simulink model "all_test"  (R2023a)
settings: Solver=VariableStepAuto  StartTime=0.0  StopTime=Tf  RelTol=1e-3
values from neighbouring files (symbols this model uses):
  vehicle_data = getVehicleDataStruct()    [main.m]
undefined symbols (not defined in the file or in its folder): input
libraries: autolibshared x5
settings Model: Creator=ashkan  LastModifiedBy=ashkan

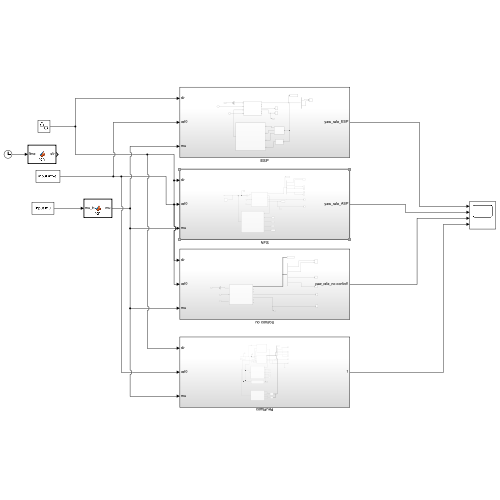
[thumbnail: Simulink's stored preview of the top-level diagram]
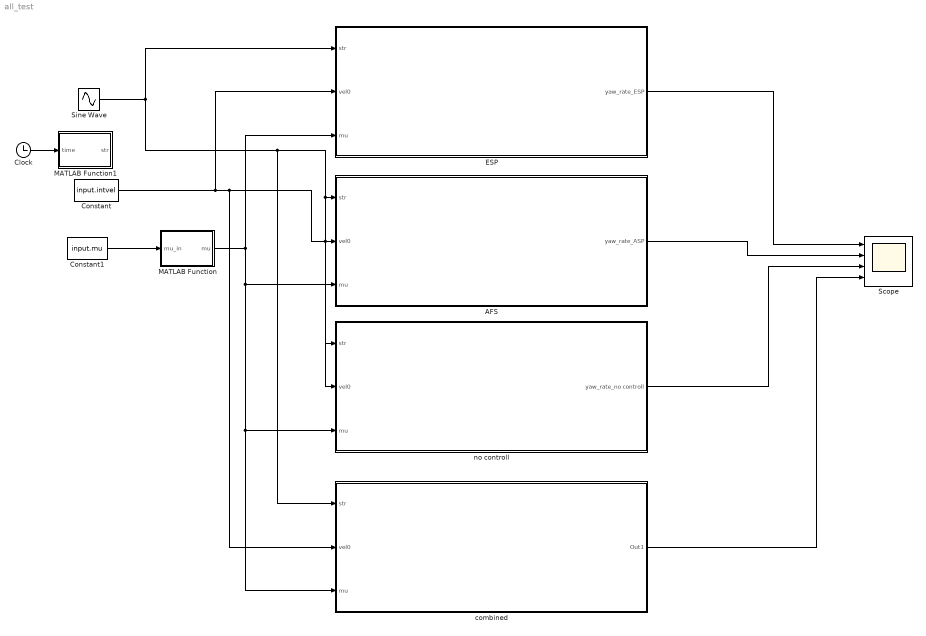
== system all_test ==
  AFS : Subsystem
  Clock : Clock
  Constant : Constant  Value=input.intvel
  Constant1 : Constant  Value=input.mu
  ESP : Subsystem
  MATLAB Function : MATLAB Function  TreatAsAtomicUnit=on
  MATLAB Function1 : MATLAB Function  TreatAsAtomicUnit=on
  Scope : Scope  NumInputPorts=4
  Sine Wave : Sin  Amplitude=input.str.amp  Frequency=input.str.freq  SampleTime=input.str.sample_time
  combined : Subsystem
  no controll : Subsystem
  wires:
  Constant/1 -> combined/2(vel0), no controll/2(vel0), AFS/2(vel0), ESP/2(vel0)
  Constant1/1 -> MATLAB Function/1(mu_in)
  Sine Wave/1 -> combined/1(str), no controll/1(str), AFS/1(str), ESP/1(str)
  MATLAB Function/1(mu) -> ESP/3(mu), AFS/3(mu), combined/3(mu), no controll/3(mu)
  ESP/1(yaw_rate_ESP) -> Scope/1
  AFS/1(yaw_rate_ASP) -> Scope/2
  no controll/1(yaw_rate_no controll) -> Scope/3
  Clock/1 -> MATLAB Function1/1(time)
  combined/1(Out1) -> Scope/4

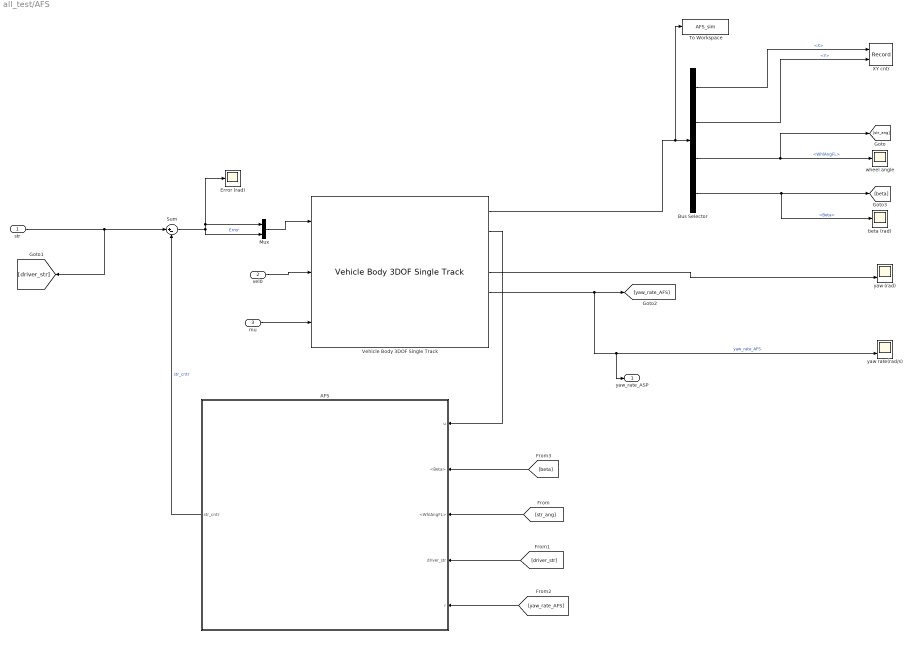
== system all_test/AFS ==
  str : Inport
  vel0 : Inport  Port=2
  mu : Inport  Port=3
  AFS : Subsystem
  Bus Selector : BusSelector  OutputSignals=InertFrm.Cg.Disp.X,InertFrm.Cg.Disp.Y,BdyFrm.FrntAxl.Steer.WhlAngFL,BdyFrm.Cg.Ang.Beta
  Error (rad) : Scope
  Mux : Mux  Inputs=2
  Sum : Sum  Inputs=|+-
  To Workspace : ToWorkspace  VariableName=AFS_sim  SaveFormat=Timeseries  SampleTime=-1
  Vehicle Body 3DOF Single Track : autolibshared/Vehicle Body 3DOF Single Track  trackMode=Dual  inputMode=External longitudinal velocity  frontSteerMode=on  rearSteerMode=off  windMode=off  muMode=on  extFMode=off  extMMode=off  htchFMode=off  htchMMode=off  extXo=off  extpsio=off  extxdoto=off  extro=off  extYo=off  extTamb=off  extydoto=off  aMode=2  NF=2  NR=2  m=vehicle_data.vehicle.m  a=vehicle_data.vehicle.Lf  b=vehicle_data.vehicle.Lr  h=vehicle_data.vehicle.hGs  dh=1  hh=0.2  X_o=0  xdot_o=0  CalphaMode=off  sigmaMode=off  d=0  hl=0  w="[vehicle_data.vehicle.Wf ,  vehicle_data.vehicle.Wr]"  Cy_f=vehicle_data.front_suspension.Ks_f  Cy_r=vehicle_data.rear_suspension.Ks_r  sigma_f=.1  sigma_r=.1  alpha_f_brk=[-.1 .1]  Cy_f_data=[-9e3 9e3]  alpha_r_brk=[-.1 .1]  Cy_r_data=[-9e3 9e3]  Y_o=0  ydot_o=0  Izz=4000  psi_o=0  r_o=0  Af=2  Cd=.3  Cl=.1  Cpm=.1  beta_w=[0 0.01:0.01:0.3]  Cs=[0 0.01:0.01:0.3]  Cym=[0 1e-6:0.01:0.3]  Pabs=101325  Tair=273  g=9.81  mu=1  xdot_tol=.01  Fznom=5000  Fxtire_sat=7e4  Fytire_sat=7e4  longOff=0  latOff=0  vertOff=0  wrapAng=off
  XY cntr : Record  FileSettingsInternal="{\"entries\":[{\"content\":{\"excelSettings\":{\"content\":{},\"type\":\"Streamout.ExcelSettings\"}},\"type\":\"Streamout.FileSettingStorage\",\"uuid\":\"\"}],\"packageUris\":[\"http:\\/\\/schema.mathworks.com\\/mf0\\/streamout_blocks\\/R2020a\"],\"version\":\"1.0\"}"  Layout=[1 1]  SignalsInternal="{\"entries\":[{\"content\":{\"signals\":[{\"content\":{\"blockPath\":[],\"dimensions\":[1],\"domain\":\"\",\"lineColor\":\"#22b573\",\"plots\":[1],\"port\":1,\"sid\":[\"\"],\"signalID\":22727,\"signalName\":\"<X>\"},\"type\":\"RecordBlkView.Signal\",\"uuid\":\"\"},{\"content\":{\"blockPath\":[],\"dimensions\":[1],\"domain\":\"\",\"lineColor\":\"#0072bd\",\"plots\":[1],\"port\":2,\"sid\":[\"\"],\"signalID\":22731,\"signalName\":\"<Y>\"},\"type\":\"RecordBlkView.Signal\",\"uuid\":\"\"}]},\"type\":\"RecordBlkView.InputSignals\",\"uuid\":\"\"}],\"packageUris\":[\"http:\\/\\/schema.mathworks.com\\/mf0\\/streamout_blocks\\/R2020a\"],\"version\":\"1.0\"}"  VisualizationBindings="{\"xyplotplugin\":{\"info\":[{\"series\":[{\"bindingParametersList\":[{\"parameter\":\"X-Axis\",\"signalID\":22727,\"signalName\":\"<X>\"},{\"parameter\":\"Y-Axis\",\"signalID\":22731,\"signalName\":\"<Y>\"}],\"seriesID\":47189}],\"subplotID\":1}]}}"  CompatibilityTag=XY
  beta (rad) : Scope
  wheel angle : Scope
  yaw (rad) : Scope  NumInputPorts=2
  yaw rate(rad/s) : Scope  NumInputPorts=2
  yaw_rate_ASP : Outport
  wires:
  Bus Selector/1 -> XY cntr/1  "<X>"
  [yaw_rate_AFS] -> AFS/5(r)
  Bus Selector/4 -> [beta], beta (rad)/1  "<Beta>"
  Bus Selector/3 -> [str_ang], wheel angle/1  "<WhlAngFL>"
  AFS/1(str_cntr) -> Sum/2  "str_cntr"
  Bus Selector/2 -> XY cntr/2  "<Y>"
  [str_ang] -> AFS/3(<WhlAngFL>)
  Vehicle Body 3DOF Single Track/5 -> [yaw_rate_AFS], yaw_rate_ASP/1, yaw rate(rad/s)/2  "yaw_rate_AFS"
  [driver_str] -> AFS/4(driver_str)
  str/1 -> [driver_str], Sum/1
  [beta] -> AFS/2(<Beta>)
  Sum/1 -> Mux/2, Mux/1, Error (rad)/1  "Error"
  Vehicle Body 3DOF Single Track/4 -> yaw (rad)/2
  Mux/1 -> Vehicle Body 3DOF Single Track/1
  Vehicle Body 3DOF Single Track/1 -> To Workspace/1, Bus Selector/1
  Vehicle Body 3DOF Single Track/2 -> AFS/1(u)
  vel0/1 -> Vehicle Body 3DOF Single Track/2
  mu/1 -> Vehicle Body 3DOF Single Track/3

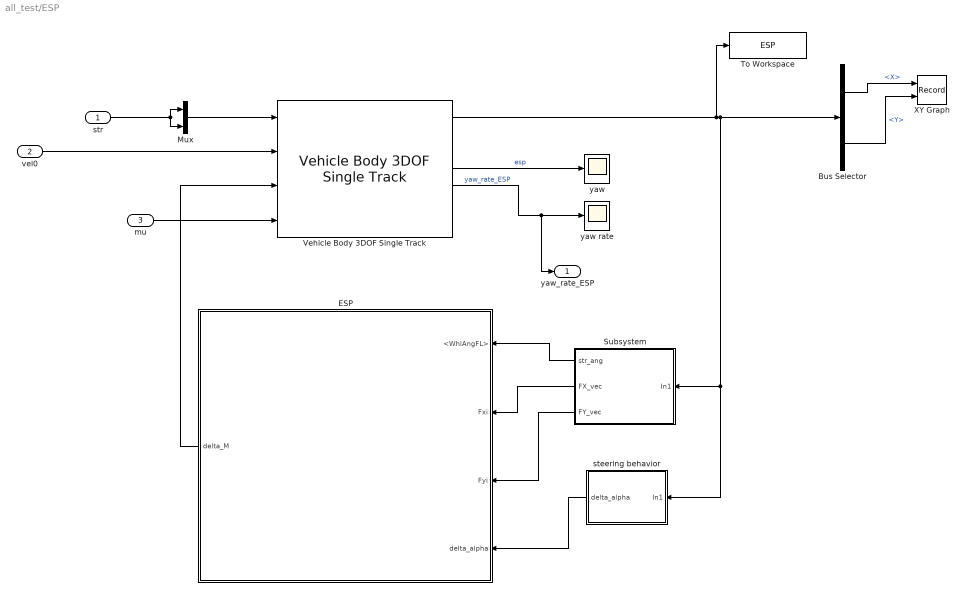
== system all_test/ESP ==
  str : Inport
  vel0 : Inport  Port=2
  mu : Inport  Port=3
  Bus Selector : BusSelector  OutputSignals=InertFrm.Cg.Disp.X,InertFrm.Cg.Disp.Y
  ESP : Subsystem
  Mux : Mux  Inputs=2
  Subsystem : Subsystem
  To Workspace : ToWorkspace  VariableName=ESP  SaveFormat=Timeseries  SampleTime=-1
  Vehicle Body 3DOF Single Track : autolibshared/Vehicle Body 3DOF Single Track  trackMode=Dual  inputMode=External longitudinal velocity  frontSteerMode=on  rearSteerMode=off  windMode=off  muMode=on  extFMode=off  extMMode=on  htchFMode=off  htchMMode=off  extXo=off  extpsio=off  extxdoto=off  extro=off  extYo=off  extTamb=off  extydoto=off  aMode=2  NF=2  NR=2  m=vehicle_data.vehicle.m  a=vehicle_data.vehicle.Lf  b=vehicle_data.vehicle.Lr  h=vehicle_data.vehicle.hGs  dh=1  hh=0.2  X_o=0  xdot_o=0  CalphaMode=off  sigmaMode=off  d=0  hl=0  w="[vehicle_data.vehicle.Wf ,  vehicle_data.vehicle.Wr]"  Cy_f=vehicle_data.front_suspension.Ks_f  Cy_r=vehicle_data.rear_suspension.Ks_r  sigma_f=.1  sigma_r=.1  alpha_f_brk=[-.1 .1]  Cy_f_data=[-9e3 9e3]  alpha_r_brk=[-.1 .1]  Cy_r_data=[-9e3 9e3]  Y_o=0  ydot_o=0  Izz=4000  psi_o=0  r_o=0  Af=2  Cd=.3  Cl=.1  Cpm=.1  beta_w=[0 0.01:0.01:0.3]  Cs=[0 0.01:0.01:0.3]  Cym=[0 1e-6:0.01:0.3]  Pabs=101325  Tair=273  g=9.81  mu=1  xdot_tol=.01  Fznom=5000  Fxtire_sat=7e4  Fytire_sat=7e4  longOff=0  latOff=0  vertOff=0  wrapAng=off
  XY Graph : Record  FileSettingsInternal="{\"entries\":[{\"content\":{\"excelSettings\":{\"content\":{},\"type\":\"Streamout.ExcelSettings\"}},\"type\":\"Streamout.FileSettingStorage\",\"uuid\":\"\"}],\"packageUris\":[\"http:\\/\\/schema.mathworks.com\\/mf0\\/streamout_blocks\\/R2020a\"],\"version\":\"1.0\"}"  Layout=[1 1]  SignalsInternal="{\"entries\":[{\"content\":{\"signals\":[{\"content\":{\"blockPath\":[],\"dimensions\":[1],\"domain\":\"\",\"lineColor\":\"#b746ff\",\"port\":1,\"sid\":[\"\"],\"signalID\":23776,\"signalName\":\"<X>\"},\"type\":\"RecordBlkView.Signal\",\"uuid\":\"\"},{\"content\":{\"blockPath\":[],\"dimensions\":[1],\"domain\":\"\",\"lineColor\":\"#64d413\",\"port\":2,\"sid\":[\"\"],\"signalID\":23780,\"signalName\":\"<Y>\"},\"type\":\"RecordBlkView.Signal\",\"uuid\":\"\"}]},\"type\":\"RecordBlkView.InputSignals\",\"uuid\":\"\"}],\"packageUris\":[\"http:\\/\\/schema.mathworks.com\\/mf0\\/streamout_blocks\\/R2020a\"],\"version\":\"1.0\"}"  VisualizationBindings="{\"xyplotplugin\":{\"info\":[{\"series\":[],\"subplotID\":1}]}}"  CompatibilityTag=XY
  steering behavior : Subsystem
  yaw : Scope
  yaw rate : Scope
  yaw_rate_ESP : Outport
  wires:
  Bus Selector/2 -> XY Graph/2  "<Y>"
  vel0/1 -> Vehicle Body 3DOF Single Track/2
  Vehicle Body 3DOF Single Track/1 -> To Workspace/1, Subsystem/1(In1), steering behavior/1(In1), Bus Selector/1
  Subsystem/2(FX_vec) -> ESP/2(Fxi)
  Subsystem/3(FY_vec) -> ESP/3(Fyi)
  Vehicle Body 3DOF Single Track/4 -> yaw/1  "esp"
  Vehicle Body 3DOF Single Track/5 -> yaw_rate_ESP/1, yaw rate/1  "yaw_rate_ESP"
  ESP/1(delta_M) -> Vehicle Body 3DOF Single Track/3
  mu/1 -> Vehicle Body 3DOF Single Track/4
  Subsystem/1(str_ang) -> ESP/1(<WhlAngFL>)
  Bus Selector/1 -> XY Graph/1  "<X>"
  str/1 -> Mux/1, Mux/2
  Mux/1 -> Vehicle Body 3DOF Single Track/1
  steering behavior/1(delta_alpha) -> ESP/4(delta_alpha)

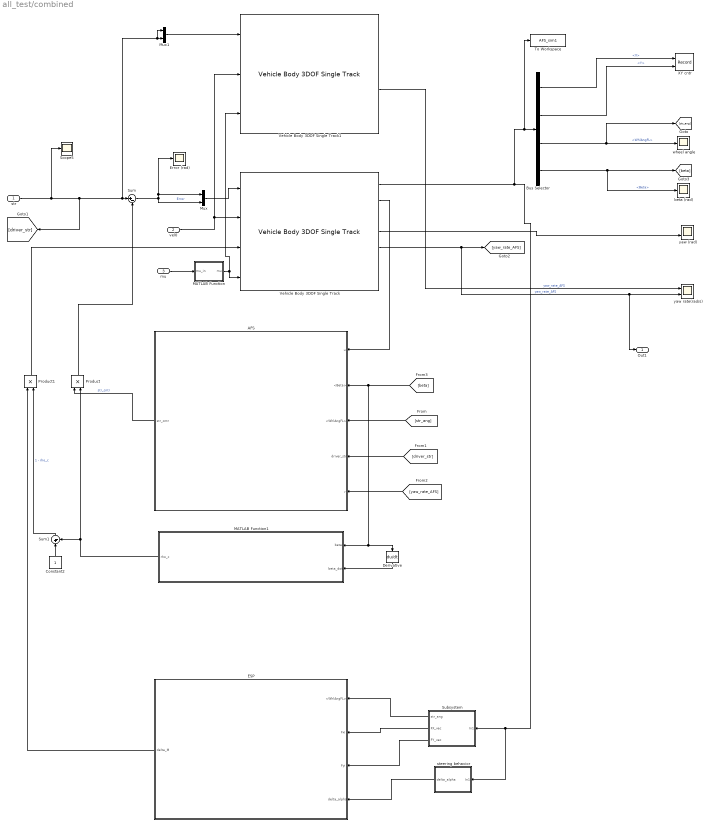
== system all_test/combined ==
  str : Inport
  vel0 : Inport  Port=2
  mu : Inport  Port=3
  AFS : Subsystem
  Bus Selector : BusSelector  OutputSignals=InertFrm.Cg.Disp.X,InertFrm.Cg.Disp.Y,BdyFrm.FrntAxl.Steer.WhlAngFL,BdyFrm.Cg.Ang.Beta
  Constant2 : Constant
  Derivative : Derivative
  ESP : Subsystem
  Error (rad) : Scope
  MATLAB Function : MATLAB Function  TreatAsAtomicUnit=on
  MATLAB Function1 : MATLAB Function  TreatAsAtomicUnit=on
  Mux : Mux  Inputs=2
  Mux1 : Mux  Inputs=2
  Product : Product
  Product1 : Product
  Scope5 : Scope
  Subsystem : Subsystem
  Sum : Sum  Inputs=|+-
  Sum1 : Sum  Inputs=|+-
  To Workspace : ToWorkspace  VariableName=AFS_sim1  SaveFormat=Timeseries  SampleTime=-1
  Vehicle Body 3DOF Single Track : autolibshared/Vehicle Body 3DOF Single Track  trackMode=Dual  inputMode=External longitudinal velocity  frontSteerMode=on  rearSteerMode=off  windMode=off  muMode=on  extFMode=off  extMMode=on  htchFMode=off  htchMMode=off  extXo=off  extpsio=off  extxdoto=off  extro=off  extYo=off  extTamb=off  extydoto=off  aMode=2  NF=2  NR=2  m=vehicle_data.vehicle.m  a=vehicle_data.vehicle.Lf  b=vehicle_data.vehicle.Lr  h=vehicle_data.vehicle.hGs  dh=1  hh=0.2  X_o=0  xdot_o=0  CalphaMode=off  sigmaMode=off  d=0  hl=0  w="[vehicle_data.vehicle.Wf ,  vehicle_data.vehicle.Wr]"  Cy_f=vehicle_data.front_suspension.Ks_f  Cy_r=vehicle_data.rear_suspension.Ks_r  sigma_f=.1  sigma_r=.1  alpha_f_brk=[-.1 .1]  Cy_f_data=[-9e3 9e3]  alpha_r_brk=[-.1 .1]  Cy_r_data=[-9e3 9e3]  Y_o=0  ydot_o=0  Izz=4000  psi_o=0  r_o=0  Af=2  Cd=.3  Cl=.1  Cpm=.1  beta_w=[0 0.01:0.01:0.3]  Cs=[0 0.01:0.01:0.3]  Cym=[0 1e-6:0.01:0.3]  Pabs=101325  Tair=273  g=9.81  mu=1  xdot_tol=.01  Fznom=5000  Fxtire_sat=7e4  Fytire_sat=7e4  longOff=0  latOff=0  vertOff=0  wrapAng=off
  Vehicle Body 3DOF Single Track1 : autolibshared/Vehicle Body 3DOF Single Track  trackMode=Dual  inputMode=External longitudinal velocity  frontSteerMode=on  rearSteerMode=off  windMode=off  muMode=on  extFMode=off  extMMode=off  htchFMode=off  htchMMode=off  extXo=off  extpsio=off  extxdoto=off  extro=off  extYo=off  extTamb=off  extydoto=off  aMode=2  NF=2  NR=2  m=vehicle_data.vehicle.m  a=vehicle_data.vehicle.Lf  b=vehicle_data.vehicle.Lr  h=vehicle_data.vehicle.hGs  dh=1  hh=0.2  X_o=0  xdot_o=0  CalphaMode=off  sigmaMode=off  d=0  hl=0  w="[vehicle_data.vehicle.Wf ,  vehicle_data.vehicle.Wr]"  Cy_f=vehicle_data.front_suspension.Ks_f  Cy_r=vehicle_data.rear_suspension.Ks_r  sigma_f=.1  sigma_r=.1  alpha_f_brk=[-.1 .1]  Cy_f_data=[-9e3 9e3]  alpha_r_brk=[-.1 .1]  Cy_r_data=[-9e3 9e3]  Y_o=0  ydot_o=0  Izz=4000  psi_o=0  r_o=0  Af=2  Cd=.3  Cl=.1  Cpm=.1  beta_w=[0 0.01:0.01:0.3]  Cs=[0 0.01:0.01:0.3]  Cym=[0 1e-6:0.01:0.3]  Pabs=101325  Tair=273  g=9.81  mu=1  xdot_tol=.01  Fznom=5000  Fxtire_sat=7e4  Fytire_sat=7e4  longOff=0  latOff=0  vertOff=0  wrapAng=off
  XY cntr : Record  FileSettingsInternal="{\"entries\":[{\"content\":{\"excelSettings\":{\"content\":{},\"type\":\"Streamout.ExcelSettings\"}},\"type\":\"Streamout.FileSettingStorage\",\"uuid\":\"\"}],\"packageUris\":[\"http:\\/\\/schema.mathworks.com\\/mf0\\/streamout_blocks\\/R2020a\"],\"version\":\"1.0\"}"  Layout=[1 1]  SignalsInternal="{\"entries\":[{\"content\":{\"signals\":[{\"content\":{\"blockPath\":[],\"dimensions\":[1],\"domain\":\"\",\"lineColor\":\"#22b573\",\"plots\":[1],\"port\":1,\"sid\":[\"\"],\"signalID\":24874,\"signalName\":\"<X>\"},\"type\":\"RecordBlkView.Signal\",\"uuid\":\"\"},{\"content\":{\"blockPath\":[],\"dimensions\":[1],\"domain\":\"\",\"lineColor\":\"#0072bd\",\"plots\":[1],\"port\":2,\"sid\":[\"\"],\"signalID\":24878,\"signalName\":\"<Y>\"},\"type\":\"RecordBlkView.Signal\",\"uuid\":\"\"}]},\"type\":\"RecordBlkView.InputSignals\",\"uuid\":\"\"}],\"packageUris\":[\"http:\\/\\/schema.mathworks.com\\/mf0\\/streamout_blocks\\/R2020a\"],\"version\":\"1.0\"}"  VisualizationBindings="{\"xyplotplugin\":{\"info\":[{\"series\":[{\"bindingParametersList\":[{\"parameter\":\"X-Axis\",\"signalID\":24874,\"signalName\":\"<X>\"},{\"parameter\":\"Y-Axis\",\"signalID\":24878,\"signalName\":\"<Y>\"}],\"seriesID\":48915}],\"subplotID\":1}]}}"  CompatibilityTag=XY
  beta (rad) : Scope
  steering behavior : Subsystem
  wheel angle : Scope
  yaw (rad) : Scope  NumInputPorts=2
  yaw rate(rad/s) : Scope  NumInputPorts=2
  Out1 : Outport
  wires:
  Vehicle Body 3DOF Single Track/1 -> steering behavior/1(In1), Subsystem/1(In1), To Workspace/1, Bus Selector/1
  Bus Selector/4 -> [beta], beta (rad)/1  "<Beta>"
  [beta] -> Derivative/1, MATLAB Function1/1(beta), AFS/2(<Beta>)
  str/1 -> [driver_str], Mux1/1, Mux1/2, Sum/1, Scope5/1
  Bus Selector/2 -> XY cntr/2  "<Y>"
  Sum1/1 -> Product1/2  "1 - rho_c"
  [yaw_rate_AFS] -> AFS/5(r)
  MATLAB Function/1(mu) -> Vehicle Body 3DOF Single Track1/3, Vehicle Body 3DOF Single Track/4
  Vehicle Body 3DOF Single Track/4 -> yaw (rad)/2
  AFS/1(str_cntr) -> Product/1  "str_cntr"
  Product1/1 -> Vehicle Body 3DOF Single Track/3
  Bus Selector/1 -> XY cntr/1  "<X>"
  Mux/1 -> Vehicle Body 3DOF Single Track/1
  Vehicle Body 3DOF Single Track/5 -> [yaw_rate_AFS], Out1/1, yaw rate(rad/s)/2  "yaw_rate_AFS"
  vel0/1 -> Vehicle Body 3DOF Single Track/2, Vehicle Body 3DOF Single Track1/2
  [driver_str] -> AFS/4(driver_str)
  Sum/1 -> Mux/2, Mux/1, Error (rad)/1  "Error"
  ESP/1(delta_M) -> Product1/1
  mu/1 -> MATLAB Function/1(mu_in)
  Vehicle Body 3DOF Single Track/2 -> AFS/1(u)
  steering behavior/1(delta_alpha) -> ESP/4(delta_alpha)
  Subsystem/2(FX_vec) -> ESP/2(Fxi)
  Subsystem/3(FY_vec) -> ESP/3(Fyi)
  Subsystem/1(str_ang) -> ESP/1(<WhlAngFL>)
  Bus Selector/3 -> [str_ang], wheel angle/1  "<WhlAngFL>"
  [str_ang] -> AFS/3(<WhlAngFL>)
  Constant2/1 -> Sum1/1
  Product/1 -> Sum/2
  Derivative/1 -> MATLAB Function1/2(beta_dot)
  MATLAB Function1/1(rho_c) -> Sum1/2, Product/2
  Mux1/1 -> Vehicle Body 3DOF Single Track1/1
  Vehicle Body 3DOF Single Track1/5 -> yaw rate(rad/s)/1  "yaw_rate_AFS"

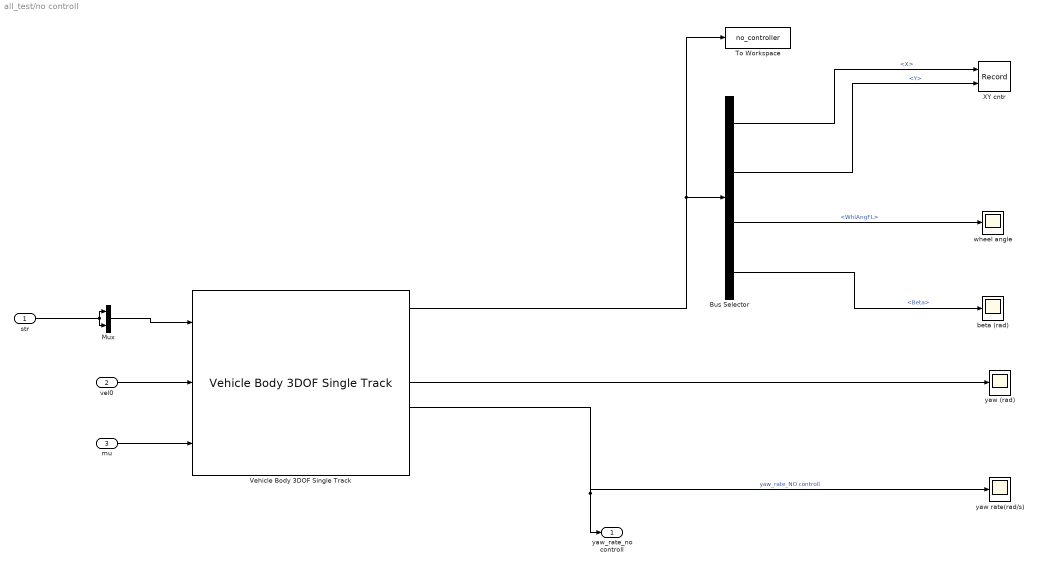
== system all_test/no controll ==
  str : Inport
  vel0 : Inport  Port=2
  mu : Inport  Port=3
  Bus Selector : BusSelector  OutputSignals=InertFrm.Cg.Disp.X,InertFrm.Cg.Disp.Y,BdyFrm.FrntAxl.Steer.WhlAngFL,BdyFrm.Cg.Ang.Beta
  Mux : Mux  Inputs=2
  To Workspace : ToWorkspace  VariableName=no_controller  SaveFormat=Timeseries  SampleTime=-1
  Vehicle Body 3DOF Single Track : autolibshared/Vehicle Body 3DOF Single Track  trackMode=Dual  inputMode=External longitudinal velocity  frontSteerMode=on  rearSteerMode=off  windMode=off  muMode=on  extFMode=off  extMMode=off  htchFMode=off  htchMMode=off  extXo=off  extpsio=off  extxdoto=off  extro=off  extYo=off  extTamb=off  extydoto=off  aMode=2  NF=2  NR=2  m=vehicle_data.vehicle.m  a=vehicle_data.vehicle.Lf  b=vehicle_data.vehicle.Lr  h=vehicle_data.vehicle.hGs  dh=1  hh=0.2  X_o=0  xdot_o=0  CalphaMode=off  sigmaMode=off  d=0  hl=0  w="[vehicle_data.vehicle.Wf ,  vehicle_data.vehicle.Wr]"  Cy_f=vehicle_data.front_suspension.Ks_f  Cy_r=vehicle_data.rear_suspension.Ks_r  sigma_f=.1  sigma_r=.1  alpha_f_brk=[-.1 .1]  Cy_f_data=[-9e3 9e3]  alpha_r_brk=[-.1 .1]  Cy_r_data=[-9e3 9e3]  Y_o=0  ydot_o=0  Izz=4000  psi_o=0  r_o=0  Af=2  Cd=.3  Cl=.1  Cpm=.1  beta_w=[0 0.01:0.01:0.3]  Cs=[0 0.01:0.01:0.3]  Cym=[0 1e-6:0.01:0.3]  Pabs=101325  Tair=273  g=9.81  mu=1  xdot_tol=.01  Fznom=5000  Fxtire_sat=7e4  Fytire_sat=7e4  longOff=0  latOff=0  vertOff=0  wrapAng=off
  XY cntr : Record  FileSettingsInternal="{\"entries\":[{\"content\":{\"excelSettings\":{\"content\":{},\"type\":\"Streamout.ExcelSettings\"}},\"type\":\"Streamout.FileSettingStorage\",\"uuid\":\"\"}],\"packageUris\":[\"http:\\/\\/schema.mathworks.com\\/mf0\\/streamout_blocks\\/R2020a\"],\"version\":\"1.0\"}"  Layout=[1 1]  SignalsInternal="{\"entries\":[{\"content\":{\"signals\":[{\"content\":{\"blockPath\":[],\"dimensions\":[1],\"domain\":\"\",\"lineColor\":\"#a2142f\",\"plots\":[1],\"port\":1,\"sid\":[\"\"],\"signalID\":25968,\"signalName\":\"<X>\"},\"type\":\"RecordBlkView.Signal\",\"uuid\":\"\"},{\"content\":{\"blockPath\":[],\"dimensions\":[1],\"domain\":\"\",\"lineColor\":\"#139fff\",\"plots\":[1],\"port\":2,\"sid\":[\"\"],\"signalID\":25972,\"signalName\":\"<Y>\"},\"type\":\"RecordBlkView.Signal\",\"uuid\":\"\"}]},\"type\":\"RecordBlkView.InputSignals\",\"uuid\":\"\"}],\"packageUris\":[\"http:\\/\\/schema.mathworks.com\\/mf0\\/streamout_blocks\\/R2020a\"],\"version\":\"1.0\"}"  VisualizationBindings="{\"xyplotplugin\":{\"info\":[{\"series\":[{\"bindingParametersList\":[{\"parameter\":\"X-Axis\",\"signalID\":25968,\"signalName\":\"<X>\"},{\"parameter\":\"Y-Axis\",\"signalID\":25972,\"signalName\":\"<Y>\"}],\"seriesID\":31368}],\"subplotID\":1}]}}"  CompatibilityTag=XY
  beta (rad) : Scope
  wheel angle : Scope
  yaw (rad) : Scope
  yaw rate(rad/s) : Scope
  yaw_rate_no controll : Outport
  wires:
  vel0/1 -> Vehicle Body 3DOF Single Track/2
  str/1 -> Mux/1, Mux/2
  Bus Selector/3 -> wheel angle/1  "<WhlAngFL>"
  Bus Selector/4 -> beta (rad)/1  "<Beta>"
  Bus Selector/1 -> XY cntr/1  "<X>"
  Bus Selector/2 -> XY cntr/2  "<Y>"
  Vehicle Body 3DOF Single Track/5 -> yaw_rate_no controll/1, yaw rate(rad/s)/1  "yaw_rate_NO controll"
  Vehicle Body 3DOF Single Track/4 -> yaw (rad)/1
  Vehicle Body 3DOF Single Track/1 -> Bus Selector/1, To Workspace/1
  Mux/1 -> Vehicle Body 3DOF Single Track/1
  mu/1 -> Vehicle Body 3DOF Single Track/3

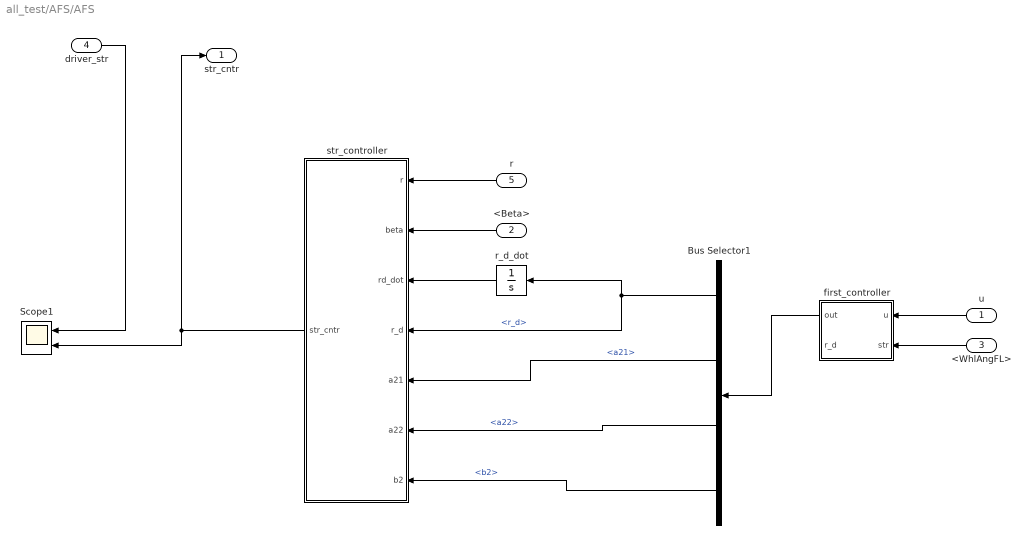
== system all_test/AFS/AFS ==
  u : Inport
  <Beta> : Inport  Port=2
  <WhlAngFL> : Inport  Port=3
  driver_str : Inport  Port=4
  r : Inport  Port=5
  Bus Selector1 : BusSelector  OutputSignals=r_d,a21,a22,b2
  Scope1 : Scope  NumInputPorts=2
  first_controller : MATLAB Function  TreatAsAtomicUnit=on
  r_d_dot : Integrator
  str_controller : MATLAB Function  TreatAsAtomicUnit=on
  str_cntr : Outport
  wires:
  driver_str/1 -> Scope1/1
  <Beta>/1 -> str_controller/2(beta)
  r/1 -> str_controller/1(r)
  first_controller/1(out) -> Bus Selector1/1
  <WhlAngFL>/1 -> first_controller/2(str)
  u/1 -> first_controller/1(u)
  Bus Selector1/2 -> str_controller/5(a21)  "<a21>"
  Bus Selector1/3 -> str_controller/6(a22)  "<a22>"
  str_controller/1(str_cntr) -> str_cntr/1, Scope1/2
  r_d_dot/1 -> str_controller/3(rd_dot)
  Bus Selector1/1 -> str_controller/4(r_d), r_d_dot/1  "<r_d>"
  Bus Selector1/4 -> str_controller/7(b2)  "<b2>"

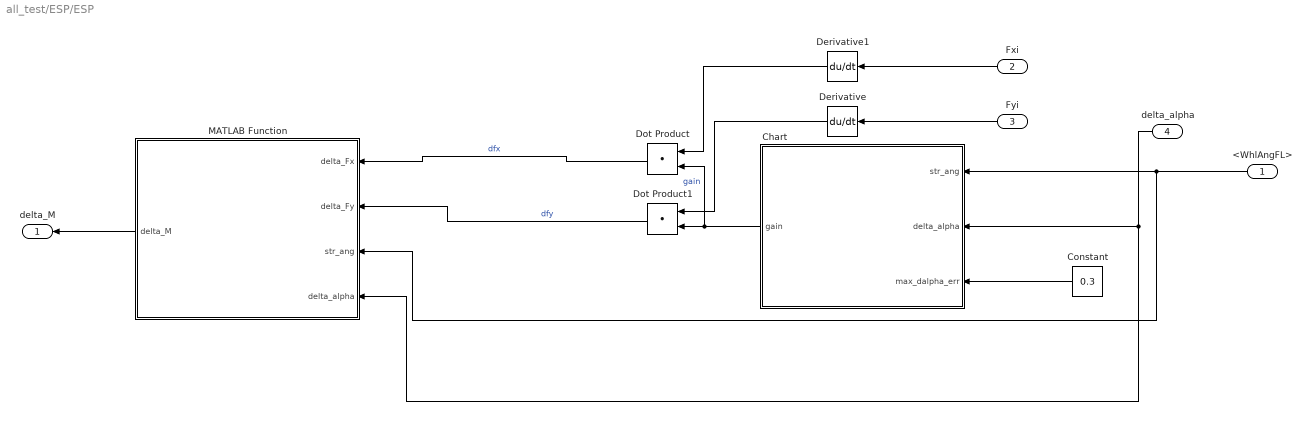
== system all_test/ESP/ESP ==
  <WhlAngFL> : Inport
  Fxi : Inport  Port=2
  Fyi : Inport  Port=3
  delta_alpha : Inport  Port=4
  Chart : Stateflow chart  TreatAsAtomicUnit=on
  Constant : Constant  Value=0.3
  Derivative : Derivative
  Derivative1 : Derivative
  Dot Product : DotProduct  OutDataTypeStr=Inherit: Inherit via internal rule
  Dot Product1 : DotProduct  OutDataTypeStr=Inherit: Inherit via internal rule
  MATLAB Function : MATLAB Function  TreatAsAtomicUnit=on
  delta_M : Outport
  wires:
  <WhlAngFL>/1 -> MATLAB Function/3(str_ang), Chart/1(str_ang)
  Constant/1 -> Chart/3(max_dalpha_err)
  Chart/1(gain) -> Dot Product1/2, Dot Product/2  "gain"
  Fxi/1 -> Derivative1/1
  Fyi/1 -> Derivative/1
  Derivative1/1 -> Dot Product/1
  Dot Product/1 -> MATLAB Function/1(delta_Fx)  "dfx"
  Derivative/1 -> Dot Product1/1
  Dot Product1/1 -> MATLAB Function/2(delta_Fy)  "dfy"
  MATLAB Function/1(delta_M) -> delta_M/1
  delta_alpha/1 -> MATLAB Function/4(delta_alpha), Chart/2(delta_alpha)

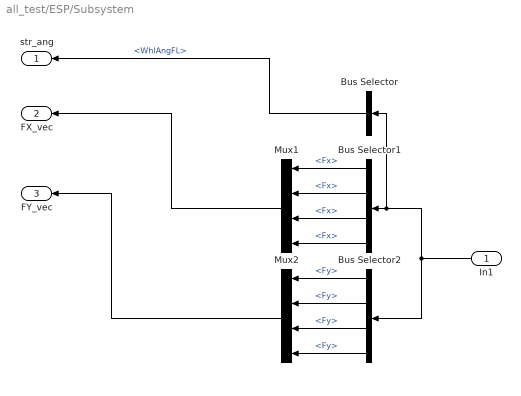
== system all_test/ESP/Subsystem ==
  In1 : Inport
  Bus Selector : BusSelector  OutputSignals=BdyFrm.FrntAxl.Steer.WhlAngFL
  Bus Selector1 : BusSelector  OutputSignals=BdyFrm.Forces.FrntAxl.Lft.Fx,BdyFrm.Forces.FrntAxl.Rght.Fx,BdyFrm.Forces.RearAxl.Lft.Fx,BdyFrm.Forces.RearAxl.Rght.Fx
  Bus Selector2 : BusSelector  OutputSignals=BdyFrm.Forces.FrntAxl.Lft.Fy,BdyFrm.Forces.FrntAxl.Rght.Fy,BdyFrm.Forces.RearAxl.Lft.Fy,BdyFrm.Forces.RearAxl.Rght.Fy
  Mux1 : Mux
  Mux2 : Mux
  str_ang : Outport
  FX_vec : Outport  Port=2
  FY_vec : Outport  Port=3
  wires:
  Mux1/1 -> FX_vec/1
  Bus Selector1/4 -> Mux1/4  "<Fx>"
  In1/1 -> Bus Selector2/1, Bus Selector/1, Bus Selector1/1
  Bus Selector2/4 -> Mux2/4  "<Fy>"
  Bus Selector1/2 -> Mux1/2  "<Fx>"
  Mux2/1 -> FY_vec/1
  Bus Selector1/3 -> Mux1/3  "<Fx>"
  Bus Selector2/3 -> Mux2/3  "<Fy>"
  Bus Selector2/1 -> Mux2/1  "<Fy>"
  Bus Selector2/2 -> Mux2/2  "<Fy>"
  Bus Selector1/1 -> Mux1/1  "<Fx>"
  Bus Selector/1 -> str_ang/1  "<WhlAngFL>"

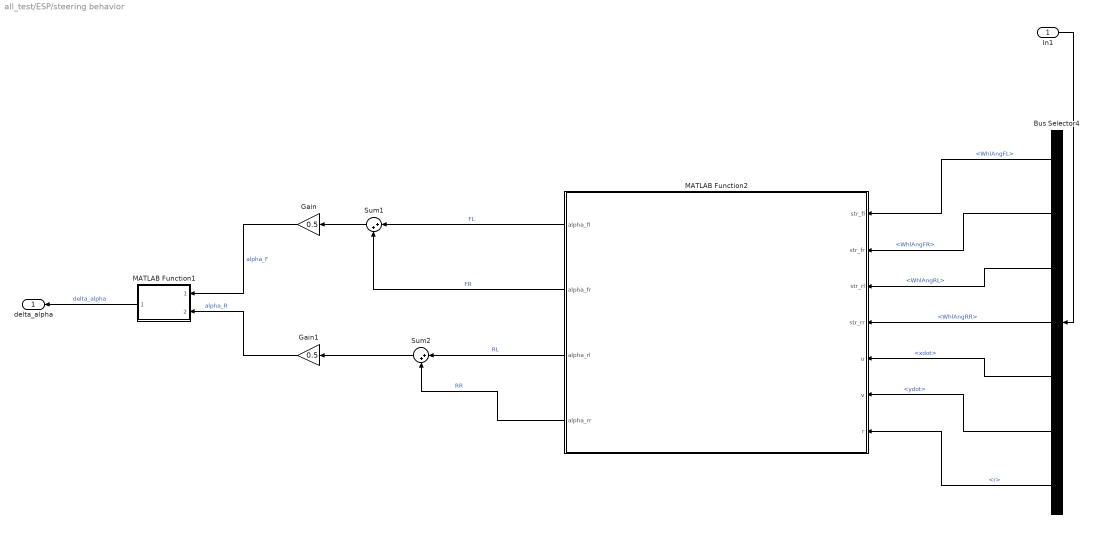
== system all_test/ESP/steering behavior ==
  In1 : Inport
  Bus Selector4 : BusSelector  OutputSignals=BdyFrm.FrntAxl.Steer.WhlAngFL,BdyFrm.FrntAxl.Steer.WhlAngFR,BdyFrm.RearAxl.Steer.WhlAngRL,BdyFrm.RearAxl.Steer.WhlAngRR,BdyFrm.Cg.Vel.xdot,BdyFrm.Cg.Vel.ydot,BdyFrm.Cg.AngVel.r
  Gain : Gain  Gain=0.5
  Gain1 : Gain  Gain=0.5
  MATLAB Function1 : MATLAB Function  TreatAsAtomicUnit=on
  MATLAB Function2 : MATLAB Function  TreatAsAtomicUnit=on
  Sum1 : Sum  Inputs=|++
  Sum2 : Sum  Inputs=|++
  delta_alpha : Outport
  wires:
  MATLAB Function1/1(delta_alpha) -> delta_alpha/1  "delta_alpha"
  In1/1 -> Bus Selector4/1
  MATLAB Function2/3(alpha_rl) -> Sum2/1  "RL"
  Sum1/1 -> Gain/1
  MATLAB Function2/2(alpha_fr) -> Sum1/2  "FR"
  MATLAB Function2/1(alpha_fl) -> Sum1/1  "FL"
  Bus Selector4/5 -> MATLAB Function2/5(u)  "<xdot>"
  Bus Selector4/3 -> MATLAB Function2/3(str_rl)  "<WhlAngRL>"
  Sum2/1 -> Gain1/1
  Gain/1 -> MATLAB Function1/1(alpha_f)  "alpha_F"
  Gain1/1 -> MATLAB Function1/2(alpha_r)  "alpha_R"
  Bus Selector4/1 -> MATLAB Function2/1(str_fl)  "<WhlAngFL>"
  Bus Selector4/6 -> MATLAB Function2/6(v)  "<ydot>"
  Bus Selector4/7 -> MATLAB Function2/7(r)  "<r>"
  MATLAB Function2/4(alpha_rr) -> Sum2/2  "RR"
  Bus Selector4/2 -> MATLAB Function2/2(str_fr)  "<WhlAngFR>"
  Bus Selector4/4 -> MATLAB Function2/4(str_rr)  "<WhlAngRR>"

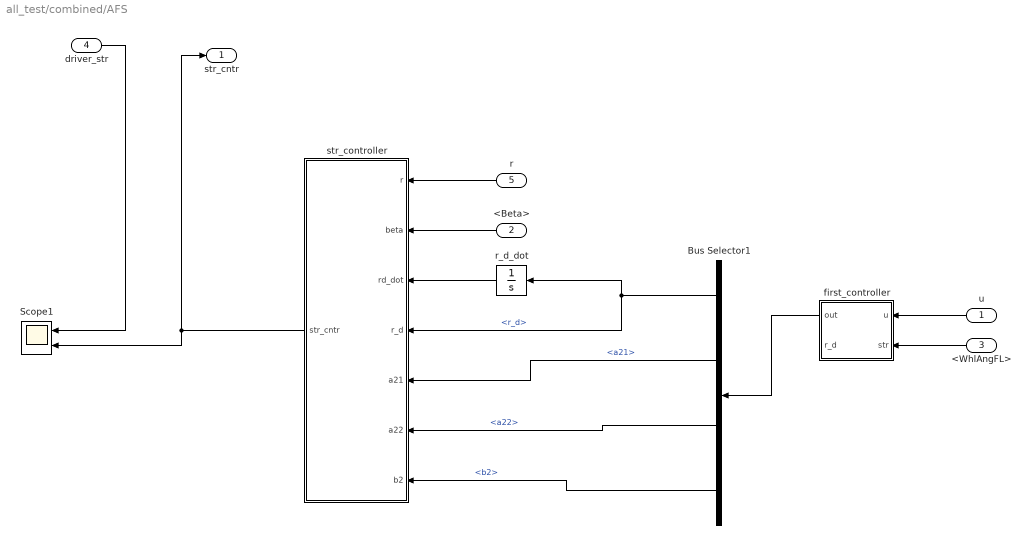
== system all_test/combined/AFS ==
  u : Inport
  <Beta> : Inport  Port=2
  <WhlAngFL> : Inport  Port=3
  driver_str : Inport  Port=4
  r : Inport  Port=5
  Bus Selector1 : BusSelector  OutputSignals=r_d,a21,a22,b2
  Scope1 : Scope  NumInputPorts=2
  first_controller : MATLAB Function  TreatAsAtomicUnit=on
  r_d_dot : Integrator
  str_controller : MATLAB Function  TreatAsAtomicUnit=on
  str_cntr : Outport
  wires:
  driver_str/1 -> Scope1/1
  <Beta>/1 -> str_controller/2(beta)
  r/1 -> str_controller/1(r)
  first_controller/1(out) -> Bus Selector1/1
  <WhlAngFL>/1 -> first_controller/2(str)
  u/1 -> first_controller/1(u)
  Bus Selector1/2 -> str_controller/5(a21)  "<a21>"
  Bus Selector1/3 -> str_controller/6(a22)  "<a22>"
  str_controller/1(str_cntr) -> str_cntr/1, Scope1/2
  r_d_dot/1 -> str_controller/3(rd_dot)
  Bus Selector1/1 -> str_controller/4(r_d), r_d_dot/1  "<r_d>"
  Bus Selector1/4 -> str_controller/7(b2)  "<b2>"

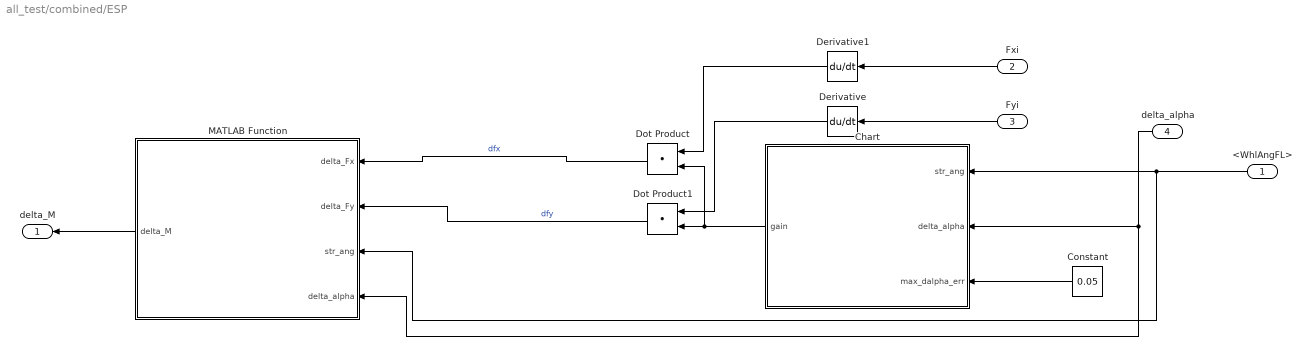
== system all_test/combined/ESP ==
  <WhlAngFL> : Inport
  Fxi : Inport  Port=2
  Fyi : Inport  Port=3
  delta_alpha : Inport  Port=4
  Chart : Stateflow chart  TreatAsAtomicUnit=on
  Constant : Constant  Value=0.05
  Derivative : Derivative
  Derivative1 : Derivative
  Dot Product : DotProduct  OutDataTypeStr=Inherit: Inherit via internal rule
  Dot Product1 : DotProduct  OutDataTypeStr=Inherit: Inherit via internal rule
  MATLAB Function : MATLAB Function  TreatAsAtomicUnit=on
  delta_M : Outport
  wires:
  <WhlAngFL>/1 -> Chart/1(str_ang), MATLAB Function/3(str_ang)
  Constant/1 -> Chart/3(max_dalpha_err)
  Chart/1(gain) -> Dot Product1/2, Dot Product/2
  Fxi/1 -> Derivative1/1
  Fyi/1 -> Derivative/1
  Derivative1/1 -> Dot Product/1
  Dot Product/1 -> MATLAB Function/1(delta_Fx)  "dfx"
  Derivative/1 -> Dot Product1/1
  Dot Product1/1 -> MATLAB Function/2(delta_Fy)  "dfy"
  MATLAB Function/1(delta_M) -> delta_M/1
  delta_alpha/1 -> Chart/2(delta_alpha), MATLAB Function/4(delta_alpha)

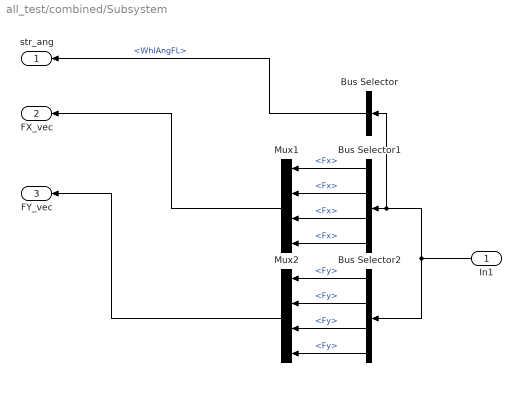
== system all_test/combined/Subsystem ==
  In1 : Inport
  Bus Selector : BusSelector  OutputSignals=BdyFrm.FrntAxl.Steer.WhlAngFL
  Bus Selector1 : BusSelector  OutputSignals=BdyFrm.Forces.FrntAxl.Lft.Fx,BdyFrm.Forces.FrntAxl.Rght.Fx,BdyFrm.Forces.RearAxl.Lft.Fx,BdyFrm.Forces.RearAxl.Rght.Fx
  Bus Selector2 : BusSelector  OutputSignals=BdyFrm.Forces.FrntAxl.Lft.Fy,BdyFrm.Forces.FrntAxl.Rght.Fy,BdyFrm.Forces.RearAxl.Lft.Fy,BdyFrm.Forces.RearAxl.Rght.Fy
  Mux1 : Mux
  Mux2 : Mux
  str_ang : Outport
  FX_vec : Outport  Port=2
  FY_vec : Outport  Port=3
  wires:
  Mux1/1 -> FX_vec/1
  Bus Selector1/4 -> Mux1/4  "<Fx>"
  In1/1 -> Bus Selector2/1, Bus Selector/1, Bus Selector1/1
  Bus Selector2/4 -> Mux2/4  "<Fy>"
  Bus Selector1/2 -> Mux1/2  "<Fx>"
  Mux2/1 -> FY_vec/1
  Bus Selector1/3 -> Mux1/3  "<Fx>"
  Bus Selector2/3 -> Mux2/3  "<Fy>"
  Bus Selector2/1 -> Mux2/1  "<Fy>"
  Bus Selector2/2 -> Mux2/2  "<Fy>"
  Bus Selector1/1 -> Mux1/1  "<Fx>"
  Bus Selector/1 -> str_ang/1  "<WhlAngFL>"

== system all_test/combined/steering behavior ==
  In1 : Inport
  Bus Selector4 : BusSelector  OutputSignals=BdyFrm.FrntAxl.Steer.WhlAngFL,BdyFrm.FrntAxl.Steer.WhlAngFR,BdyFrm.RearAxl.Steer.WhlAngRL,BdyFrm.RearAxl.Steer.WhlAngRR,BdyFrm.Cg.Vel.xdot,BdyFrm.Cg.Vel.ydot,BdyFrm.Cg.AngVel.r
  Gain : Gain  Gain=0.5
  Gain1 : Gain  Gain=0.5
  MATLAB Function1 : MATLAB Function  TreatAsAtomicUnit=on
  MATLAB Function2 : MATLAB Function  TreatAsAtomicUnit=on
  Sum1 : Sum  Inputs=|++
  Sum2 : Sum  Inputs=|++
  delta_alpha : Outport
  wires:
  MATLAB Function1/1(delta_alpha) -> delta_alpha/1  "delta_alpha"
  In1/1 -> Bus Selector4/1
  MATLAB Function2/3(alpha_rl) -> Sum2/1  "RL"
  Sum1/1 -> Gain/1
  MATLAB Function2/2(alpha_fr) -> Sum1/2  "FR"
  MATLAB Function2/1(alpha_fl) -> Sum1/1  "FL"
  Bus Selector4/5 -> MATLAB Function2/5(u)  "<xdot>"
  Bus Selector4/3 -> MATLAB Function2/3(str_rl)  "<WhlAngRL>"
  Sum2/1 -> Gain1/1
  Gain/1 -> MATLAB Function1/1(alpha_f)  "alpha_F"
  Gain1/1 -> MATLAB Function1/2(alpha_r)  "alpha_R"
  Bus Selector4/1 -> MATLAB Function2/1(str_fl)  "<WhlAngFL>"
  Bus Selector4/6 -> MATLAB Function2/6(v)  "<ydot>"
  Bus Selector4/7 -> MATLAB Function2/7(r)  "<r>"
  MATLAB Function2/4(alpha_rr) -> Sum2/2  "RR"
  Bus Selector4/2 -> MATLAB Function2/2(str_fr)  "<WhlAngFR>"
  Bus Selector4/4 -> MATLAB Function2/4(str_rr)  "<WhlAngRR>"

== stateflow chart all_test/ESP/ESP/Chart ==
  state ESP_ON
    state FRONT_WHEEL
      state FRONT_LEFT
        gain = [1 0 0 0];
      state FRONT_RIGHT
        gain = [0 1 0 0] ;
      (junction 36) -> FRONT_LEFT [order 2] : [str_ang >0]
      (junction 36) -> FRONT_RIGHT [order 1] : [str_ang <     0]
      FRONT_RIGHT -> (junction 36)
      FRONT_LEFT -> (junction 36)
    state REAR_WHEEL
      state REAR_LEFT
        gain = [0 0 1 0];
      state REAR_RIGHT
        gain = [0 0 0 1];
      (junction 38) -> REAR_LEFT [order 1] : [str_ang > 0]
      (junction 38) -> REAR_RIGHT [order 2] : [str_ang > 0]
      REAR_RIGHT -> (junction 38)
      REAR_LEFT -> (junction 38)
    (junction 31) -> (junction 36) [order 1] : [delta_alpha > 0 ]
    FRONT_WHEEL -> (junction 31)
    REAR_WHEEL -> (junction 31)
    (junction 31) -> (junction 38) [order 2] : [delta_alpha < 0]
  state ESP_OFF
    gain = [0 0 0 0]   ;
  (default) -> ESP_OFF
  ESP_OFF -> (junction 31) : [ abs(delta_alpha) > max_dalpha_err + 0.1   ]
  ESP_ON -> ESP_OFF : [abs(delta_alpha  ) < max_dalpha_err - 0.1]
  data: str_ang input; delta_alpha input; max_dalpha_err input; gain output

== matlab function all_test/ESP/steering behavior/MATLAB Function1 ==
  data: alpha_f input; delta_alpha output; alpha_r input
function delta_alpha = fcn(alpha_f , alpha_r)

delta_alpha = alpha_r - alpha_f;

== matlab function all_test/MATLAB Function1 ==
  data: time input; str output
function str = fcn(time)

    if time < 5
        str = 0;
    elseif time >= 5 && time < 6
        str = 1;
    elseif time >= 6 && time <15
        str = 0;
    elseif time >= 15 && time <16.6
        str = -1;
    else
        str = 0;
    end

end

== matlab function all_test/combined/AFS/first_controller ==
  data: out output Bus: out_rd_bus; u input; str input; vehicle_data parameter; r_d output
function [out, r_d] = r_d(u , str, vehicle_data)


% here is some simplified parameters :)
   m = vehicle_data.vehicle.m;
   a = vehicle_data.vehicle.Lf;
   b = vehicle_data.vehicle.Lr;
   izz = vehicle_data.vehicle.i_zz;
   g = vehicle_data.vehicle.g;
   L = vehicle_data.vehicle.L;
   mu = vehicle_data.AFS.mu;  % --> should come from scenario
   Caf = vehicle_data.front_suspension.Ks_f ;
   Car = vehicle_data.rear_suspension.Ks_r;
   
   
% lets calculate some live parameters!!! _|_
    
   r_up_lim = 0.85 * abs(mu*g / u);
   r_ss = (2*L*Caf*Car*u)/(2*Car*Caf*L^2 - m*u^2*(a*Caf - b*Car)) * str;
   r_d = min(r_ss , r_up_lim)* sign(str);
 
   a11 = (-2*Caf - 2*Car)/(m * u);
   a12 = -1 + (2*Car*b - 2*Caf*a)/(m * u^2);
   a21 = (2*Car*b - 2*Caf*a)/izz;
   a22 = (-2*Caf*a^2 - 2*Car*b^2)/(izz * u);
   b1 = (2*Caf)/(m * u);
   b2 = (2 * Caf * a)/izz;

% outputs
   out.a11 = a11;
   out.a21 = a21;
   out.a12 = a12;
   out.a22 = a22;
   out.b1 = b1;
   out.b2 = b2;
   out.r_d = r_d;

end

== matlab function all_test/combined/AFS/str_controller ==
  data: r input; beta input; rd_dot input; r_d input; a21 input; str_cntr output; a22 input; b2 input; vehicle_data parameter
function str_cntr = str_controller(r, beta , rd_dot , r_d , a21 , a22 , b2, vehicle_data)

%    lambda = AFS.lambda;
    s = r - r_d;
    lambda = vehicle_data.AFS.lambda;
    X      = vehicle_data.AFS.X;
    str_cntr = ((1/b2) * (-a21*beta - a22*r + rd_dot - lambda*(s))) - sign(s)*X;


end

== stateflow chart all_test/combined/ESP/Chart ==
  state ESP_ON
    state FRONT_WHEEL
      state FRONT_LEFT
        gain = [1 0 0 0];
      state FRONT_RIGHT
        gain = [0 1 0 0] ;
      (junction 36) -> FRONT_LEFT [order 2] : [str_ang >0]
      (junction 36) -> FRONT_RIGHT [order 1] : [str_ang <     0]
      FRONT_RIGHT -> (junction 36)
      FRONT_LEFT -> (junction 36)
    state REAR_WHEEL
      state REAR_LEFT
        gain = [0 0 1 0];
      state REAR_RIGHT
        gain = [0 0 0 1];
      (junction 38) -> REAR_LEFT [order 1] : [str_ang > 0]
      (junction 38) -> REAR_RIGHT [order 2] : [str_ang > 0]
      REAR_RIGHT -> (junction 38)
      REAR_LEFT -> (junction 38)
    (junction 31) -> (junction 36) [order 1] : [delta_alpha > 0 ]
    FRONT_WHEEL -> (junction 31)
    REAR_WHEEL -> (junction 31)
    (junction 31) -> (junction 38) [order 2] : [delta_alpha < 0]
  state ESP_OFF
    gain = [0 0 0 0]   ;
  (default) -> ESP_OFF
  ESP_OFF -> (junction 31) : [ abs(delta_alpha) > max_dalpha_err + 0.1   ]
  ESP_ON -> ESP_OFF : [abs(delta_alpha  ) < max_dalpha_err - 0.1]
  data: str_ang input; delta_alpha input; max_dalpha_err input; gain output

== matlab function all_test/combined/ESP/MATLAB Function ==
  data: delta_Fx input; delta_M output; delta_Fy input; str_ang input; delta_alpha input; vehicle_data parameter
function delta_M   = yaw_moment_diff(delta_Fx , delta_Fy ,  str_ang , delta_alpha , vehicle_data)

    a = vehicle_data.vehicle.Lf;
    b = vehicle_data.vehicle.Lr;
    L = vehicle_data.vehicle.L;
    Tw = vehicle_data.vehicle.Wf;

    if delta_alpha > 0      % over steering

    
        delta_Mz = (delta_Fx*(0.5*Tw*cos(str_ang) + a*sin(str_ang))) - (delta_Fy * (a*cos(str_ang) - 0.5*Tw*sin(str_ang)));

        
    elseif delta_alpha < 0  % under steering

        
        delta_Mz = (delta_Fx * 0.5*Tw) - (delta_Fy * b);

    else    % natural steering
        delta_Mz = 0;

    end

    delta_Mx = 0;

    delta_My = 0;

    delta_M = [delta_Mx , delta_My , delta_Mz];

end

== matlab function all_test/combined/MATLAB Function ==
  data: mu_in input; mu output
function mu = fcn(mu_in)

mu = mu_in*ones(2);

== matlab function all_test/combined/MATLAB Function1 ==
  data: beta input; rho_c output; beta_dot input
function rho_c = fcn( beta , beta_dot )

    k1 = 0;
    k2 = 10;
    b1 = 3;
    b2 = 9;
    cond = abs(k1*beta_dot + k2*beta);

    if cond < b1
        rho_c = 1;
    elseif cond >= b1 && cond <= b2
        rho_c = (b2 - cond)/(b2-b1);
    else
        rho_c = 0;
    end



end

== matlab function all_test/combined/steering behavior/MATLAB Function1 ==
  data: alpha_f input; delta_alpha output; alpha_r input
function delta_alpha = fcn(alpha_f , alpha_r)

delta_alpha = alpha_r - alpha_f;

== matlab function all_test/combined/steering behavior/MATLAB Function2 ==
  data: str_fl input; str_fr input; str_rl input; str_rr input; u input; alpha_fl output; v input; r input; alpha_fr output; alpha_rl output; alpha_rr output; vehicle_data parameter
function [alpha_fl , alpha_fr , alpha_rl , alpha_rr] = fcn(str_fl , str_fr , str_rl , str_rr , u , v , r , vehicle_data)


    a = vehicle_data.vehicle.Lf;
    b = vehicle_data.vehicle.Lr;
    Tw = vehicle_data.vehicle.Wf;
    
    alpha_fl = str_fl - atan((v+ a*r )/(u + 0.5*Tw*r ));
    alpha_fr = str_fr - atan((v+ a*r )/(u - 0.5*Tw*r ));
    alpha_rl = str_rl + atan((b*r - v )/(u + 0.5*Tw*r ));
    alpha_rr = str_rr + atan((b*r - v )/(u - 0.5*Tw*r ));


end

== matlab function all_test/ESP/steering behavior/MATLAB Function2 ==
  data: str_fl input; str_fr input; str_rl input; str_rr input; u input; alpha_fl output; v input; r input; alpha_fr output; alpha_rl output; alpha_rr output; vehicle_data parameter
function [alpha_fl , alpha_fr , alpha_rl , alpha_rr] = fcn(str_fl , str_fr , str_rl , str_rr , u , v , r , vehicle_data)


    a = vehicle_data.vehicle.Lf;
    b = vehicle_data.vehicle.Lr;
    Tw = vehicle_data.vehicle.Wf;
    
    alpha_fl = str_fl - atan((v+ a*r )/(u + 0.5*Tw*r ));
    alpha_fr = str_fr - atan((v+ a*r )/(u - 0.5*Tw*r ));
    alpha_rl = str_rl + atan((b*r - v )/(u + 0.5*Tw*r ));
    alpha_rr = str_rr + atan((b*r - v )/(u - 0.5*Tw*r ));


end

== matlab function all_test/MATLAB Function ==
  data: mu_in input; mu output
function mu = fcn(mu_in)

mu = mu_in*ones(2);

== matlab function all_test/ESP/ESP/MATLAB Function ==
  data: delta_Fx input; delta_M output; delta_Fy input; str_ang input; delta_alpha input; vehicle_data parameter
function delta_M   = yaw_moment_diff(delta_Fx , delta_Fy ,  str_ang , delta_alpha , vehicle_data)

    a = vehicle_data.vehicle.Lf;
    b = vehicle_data.vehicle.Lr;
    L = vehicle_data.vehicle.L;
    Tw = vehicle_data.vehicle.Wf;

    if delta_alpha > 0      % over steering

    
        delta_Mz = (delta_Fx*(0.5*Tw*cos(str_ang) + a*sin(str_ang))) - (delta_Fy * (a*cos(str_ang) - 0.5*Tw*sin(str_ang)));

        
    elseif delta_alpha < 0  % under steering

        
        delta_Mz = (delta_Fx * 0.5*Tw) - (delta_Fy * b);

    else    % natural steering
        delta_Mz = 0;

    end

    delta_Mx = 0;

    delta_My = 0;

    delta_M = [delta_Mx , delta_My , delta_Mz];

end

== matlab function all_test/AFS/AFS/first_controller ==
  data: out output Bus: out_rd_bus; u input; str input; vehicle_data parameter; r_d output
function [out, r_d] = r_d(u , str, vehicle_data)


% here is some simplified parameters :)
   m = vehicle_data.vehicle.m;
   a = vehicle_data.vehicle.Lf;
   b = vehicle_data.vehicle.Lr;
   izz = vehicle_data.vehicle.i_zz;
   g = vehicle_data.vehicle.g;
   L = vehicle_data.vehicle.L;
   mu = vehicle_data.AFS.mu;  % --> should come from scenario
   Caf = vehicle_data.front_suspension.Ks_f ;
   Car = vehicle_data.rear_suspension.Ks_r;
   
   
% lets calculate some live parameters!!! _|_
    
   r_up_lim = 0.85 * abs(mu*g / u);
   r_ss = (2*L*Caf*Car*u)/(2*Car*Caf*L^2 - m*u^2*(a*Caf - b*Car)) * str;
   r_d = min(r_ss , r_up_lim)* sign(str);
 
   a11 = (-2*Caf - 2*Car)/(m * u);
   a12 = -1 + (2*Car*b - 2*Caf*a)/(m * u^2);
   a21 = (2*Car*b - 2*Caf*a)/izz;
   a22 = (-2*Caf*a^2 - 2*Car*b^2)/(izz * u);
   b1 = (2*Caf)/(m * u);
   b2 = (2 * Caf * a)/izz;

% outputs
   out.a11 = a11;
   out.a21 = a21;
   out.a12 = a12;
   out.a22 = a22;
   out.b1 = b1;
   out.b2 = b2;
   out.r_d = r_d;

end

== matlab function all_test/AFS/AFS/str_controller ==
  data: r input; beta input; rd_dot input; r_d input; a21 input; str_cntr output; a22 input; b2 input; vehicle_data parameter
function str_cntr = str_controller(r, beta , rd_dot , r_d , a21 , a22 , b2, vehicle_data)

%    lambda = AFS.lambda;
    s = r - r_d;
    lambda = vehicle_data.AFS.lambda;
    X      = vehicle_data.AFS.X;
    str_cntr = ((1/b2) * (-a21*beta - a22*r + rd_dot - lambda*(s))) - sign(s)*X;


end
